simulink model "H175_Anode_Integration"  (R2023a)
settings: Solver=VariableStepAuto  StartTime=0.0  StopTime=80  RelTol=1e-3
values from neighbouring files (symbols this model uses):
  anode_tube_D = 0.01    [All_Properties.mat]    (also in anode_subsystem_parameters.m; environment_parameters.m)
  D = 0.01    [All_Properties.mat]    (also in anode_subsystem_parameters.m)
  densityHydrogen = 0.0899    [All_Properties.mat]    (also in Valve_Init.m; anode_subsystem_parameters.m)
  Kv_VL6112 = 0.8    [All_Properties.mat]    (also in anode_subsystem_parameters.m)
  N2_T = [-56.55 -50 -40 -30 -20 -10 -5 -4 -3 -2 -1 0 ... (52 elements, 1x52)]    [All_Properties.mat]    (also in anode_subsystem_parameters.m = [-56.55 -50 -40 -30 -20 -10 -5 -4 -3 -2 -1 0 1 2 3 4 5 10 20; environment_parameters.m = [-56.55, -50:10:-10, -5:1:5, 10:10:350]; stack_model_harness_parameters.m = [-56.55, -50:10:-10, -5:1:5, 10:10:350])
  p_range = 0.005    [All_Properties.mat]    (also in anode_subsystem_parameters.m)
  r_max = 0.2    [All_Properties.mat]    (also in anode_subsystem_parameters.m)
  r_min = 0.0001    [All_Properties.mat]    (also in anode_subsystem_parameters.m)
  responseTimeValve = 0.013    [All_Properties.mat]    (also in anode_subsystem_parameters.m)
libraries: fl_lib x75, nesl_utility x39, SimscapeFluids_lib x1
(part 2 of 2)

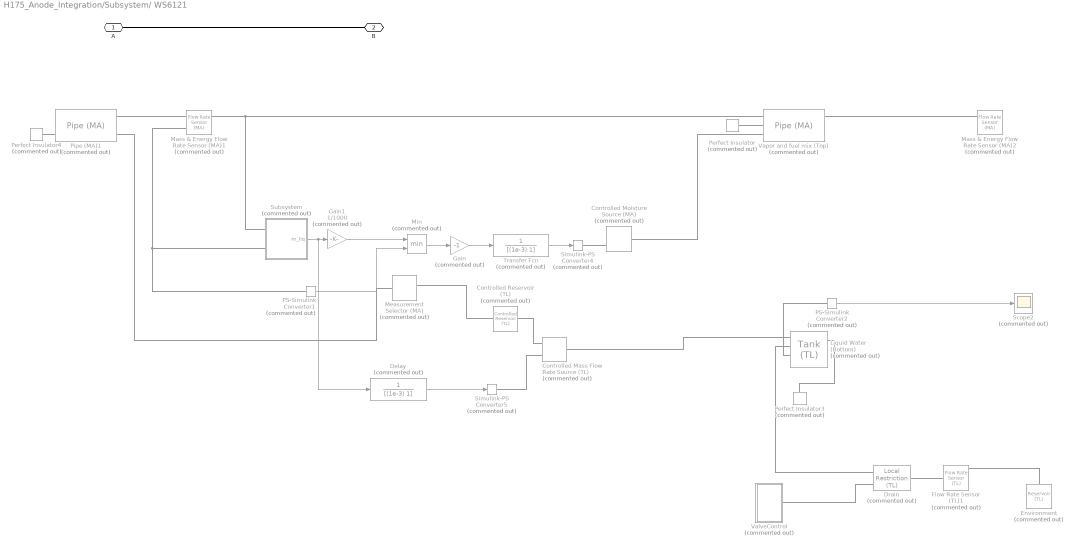
== system H175_Anode_Integration/Subsystem/ WS6121 ==
  Controlled Mass Flow Rate Source (TL) : fl_lib/Thermal Liquid/Sources/Controlled Mass Flow Rate Source (TL)  Commented=on  power_spec=foundation.enum.power_spec.isentropic  area=0.01 m^2
      settings: InternalSimscapePortConfiguration="{\"Bottom\":[],\"Left\":[{\"id\":\"A\",\"label\":\"A\",\"type\":\"foundation.thermal_liquid.thermal_liquid\"},{\"id\":\"M\",\"label\":\"M\",\"type\":\"input\"}],\"Right\":[{\"id\":\"B\",\"label\":\"B\",\"type\":\"foundation.thermal_liquid.thermal_liquid\"}],\"Top\":[]}"
  Controlled Moisture Source (MA) : fl_lib/Moist Air/Sources/Moisture & Trace Gas Sources/Controlled Moisture Source (MA)  Commented=on  moisture_source_spec=foundation.enum.moisture_source_spec.liquid  Phi_S_specify=off  Phi_S_priority=None  Phi_S=0 kW  Phi_S_nominal_specify=off  Phi_S_nominal_unit=kW  Phi_S_nominal_value=1  mdot_w_S_specify=off  mdot_w_S_priority=None  mdot_w_S=0 kg/s  mdot_w_S_nominal_specify=off  mdot_w_S_nominal_unit=kg/s  mdot_w_S_nominal_value=1
      settings: InternalSimscapePortConfiguration="{\"Bottom\":[],\"Left\":[{\"id\":\"S\",\"label\":\"S\",\"type\":\"foundation.moist_air.moist_air_source\"}],\"Right\":[{\"id\":\"M\",\"label\":\"M\",\"type\":\"input\"},{\"id\":\"T\",\"label\":\"T\",\"type\":\"input\"}],\"Top\":[]}"
  Controlled Reservoir (TL) : fl_lib/Thermal Liquid/Elements/Controlled Reservoir (TL)  Commented=on  pressure_spec=foundation.enum.pressure_spec.atmospheric  reservoir_pressure=0.101325 MPa  area=0.01 m^2
      settings: InternalSimscapePortConfiguration="{\"Bottom\":[],\"Left\":[{\"id\":\"A\",\"label\":\"A\",\"type\":\"foundation.thermal_liquid.thermal_liquid\"}],\"Right\":[{\"id\":\"T_in\",\"label\":\"T\",\"type\":\"input\"}],\"Top\":[]}"
  Delay : TransferFcn  Commented=on  Denominator=[(1e-3) 1]
  Drain : fl_lib/Thermal Liquid/Elements/Local Restriction (TL)  Commented=on  restriction_type=foundation.enum.restriction_type.variable  restriction_area=0.001 m^2  min_area=0.00001e-6 m^2  max_area=4.75e-6 m^2  area=0.00358 m^2  Cd=0.32  Re_c=150  pressure_recovery=simscape.enum.onoff.off
      settings: InternalSimscapePortConfiguration="{\"Bottom\":[],\"Left\":[{\"id\":\"A\",\"label\":\"A\",\"type\":\"foundation.thermal_liquid.thermal_liquid\"},{\"id\":\"area_in\",\"label\":\"AR\",\"type\":\"input\"}],\"Right\":[{\"id\":\"B\",\"label\":\"B\",\"type\":\"foundation.thermal_liquid.thermal_liquid\"}],\"Top\":[]}"
  Environment : fl_lib/Thermal Liquid/Elements/Reservoir (TL)  Commented=on  pressure_spec=foundation.enum.pressure_spec.atmospheric  reservoir_pressure=0.101325 MPa  reservoir_temperature=293.15 K  area=0.01 m^2
  Flow Rate Sensor (TL)1 : fl_lib/Thermal Liquid/Sensors/Flow Rate Sensor (TL)  Commented=on  mass_flow_measure=true  volumetric_flow_measure=false  energy_flow_measure=true
      settings: InternalSimscapePortConfiguration="{\"Bottom\":[{\"id\":\"PHI\",\"label\":\"φ\",\"type\":\"output\"}],\"Left\":[{\"id\":\"A\",\"label\":\"A\",\"type\":\"foundation.thermal_liquid.thermal_liquid\"}],\"Right\":[{\"id\":\"B\",\"label\":\"B\",\"type\":\"foundation.thermal_liquid.thermal_liquid\"},{\"id\":\"M\",\"label\":\"M\",\"type\":\"output\"}],\"Top\":[]}"
  Gain : Gain  Commented=on  Gain=-1
  Gain1 : Gain  Commented=on  Gain=1/1000
  "Liquid Water (Bottom) " : SimscapeFluids_lib/Thermal Liquid/Tanks & Accumulators/Tank (TL)  Commented=on  num_inlet=fluids.thermal_liquid.tanks_accumulators.enum.NumInlet.Two  pressure_spec=foundation.enum.pressure_spec.atmospheric  tank_pressure=0.101325 MPa  volume_spec=fluids.thermal_liquid.tanks_accumulators.enum.TankVolumeSpec.Constant  tank_area=0.0003 m^2  level_TLU=[0, 3, 5] m  volume_TLU=[0, 4, 6] m^3  inlet_height_A=0.00002 m  inlet_area_A=0.00002 m^2  inlet_heights_AB=[.1, .1] m  inlet_areas_AB=[.01, .01] m^2  inlet_heights_ABC=[.1, .1, .1] m  inlet_areas_ABC=[.01, .01, .01] m^2  inlet_heights_ABCD=0.1 * ones(1, 4) m  inlet_areas_ABCD=0.01 * ones(1, 4) m^2  inlet_heights_ABCDE=0.1 * ones(1, 5) m  inlet_areas_ABCDE=0.01 * ones(1, 5) m^2  inlet_heights_ABCDEF=0.1 * ones(1, 6) m  inlet_areas_ABCDEF=0.01 * ones(1, 6) m^2  level_check=simscape.enum.assert.action.error  capacity_check=simscape.enum.assert.action.warn  max_capacity=0.0003 m^3  g=9.81 m/s^2  level_specify=off  level_priority=High  level=5 m  level_nominal_specify=off  level_nominal_unit=m  level_nominal_value=1  volume_specify=off  volume_priority=None  volume=5 m^3  volume_nominal_specify=off  volume_nominal_unit=m^3  volume_nominal_value=1  mass_specify=off  mass_priority=None  mass=5000 kg  mass_nominal_specify=off  mass_nominal_unit=kg  mass_nominal_value=1  T_I_specify=off  T_I_priority=High  T_I=293.15 K  T_I_nominal_specify=off  T_I_nominal_unit=K  T_I_nominal_value=1
      settings: InternalSimscapePortConfiguration="{\"Bottom\":[{\"id\":\"H\",\"label\":\"H\",\"type\":\"foundation.thermal.thermal\"},{\"id\":\"T_out\",\"label\":\"T\",\"type\":\"output\"}],\"Left\":[{\"id\":\"A\",\"label\":\"A\",\"type\":\"foundation.thermal_liquid.thermal_liquid\"},{\"id\":\"B\",\"label\":\"B\",\"type\":\"foundation.thermal_liquid.thermal_liquid\"}],\"Right\":[],\"Top\":[{\"id\":\"V_out\",\"label\":\"V\",\"type\":\"output\"},{\"id\":\"L_out\",\"label\":\"L\",\"type\":\"output\"}]}"
  Mass & Energy Flow Rate Sensor (MA)1 : fl_lib/Moist Air/Sensors/Flow Rate Sensor (MA)  Commented=on  mass_flow_measure=true  volumetric_flow_measure=false  volumetric_flow_conditions=foundation.enum.volumetric_flow_conditions.actual  p_std=0.101325 MPa  T_std=20 degC  RH_std=0.65  energy_flow_measure=false  vapor_flow_measure=true  gas_flow_measure=false
      settings: InternalSimscapePortConfiguration="{\"Bottom\":[],\"Left\":[{\"id\":\"A\",\"label\":\"A\",\"type\":\"foundation.moist_air.moist_air\"},{\"id\":\"Mw\",\"label\":\"Mw\",\"type\":\"output\"}],\"Right\":[{\"id\":\"B\",\"label\":\"B\",\"type\":\"foundation.moist_air.moist_air\"},{\"id\":\"M\",\"label\":\"M\",\"type\":\"output\"}],\"Top\":[]}"
  Mass & Energy Flow Rate Sensor (MA)2 : fl_lib/Moist Air/Sensors/Flow Rate Sensor (MA)  Commented=on  mass_flow_measure=true  volumetric_flow_measure=false  volumetric_flow_conditions=foundation.enum.volumetric_flow_conditions.actual  p_std=0.101325 MPa  T_std=20 degC  RH_std=0.65  energy_flow_measure=false  vapor_flow_measure=true  gas_flow_measure=false
      settings: InternalSimscapePortConfiguration="{\"Bottom\":[],\"Left\":[{\"id\":\"A\",\"label\":\"A\",\"type\":\"foundation.moist_air.moist_air\"},{\"id\":\"Mw\",\"label\":\"Mw\",\"type\":\"output\"}],\"Right\":[{\"id\":\"B\",\"label\":\"B\",\"type\":\"foundation.moist_air.moist_air\"},{\"id\":\"M\",\"label\":\"M\",\"type\":\"output\"}],\"Top\":[]}"
  Measurement Selector (MA) : fl_lib/Moist Air/Sensors/Measurement Selector (MA)  Commented=on  moisture_spec=foundation.enum.moisture_spec.relative_humidity  trace_gas_spec=foundation.enum.trace_gas_spec.mass_fraction
  Min : MinMax  Commented=on  Inputs=2
  PS-Simulink Converter1 : nesl_utility/PS-Simulink Converter  Commented=on  PhysicalDomain=network_engine_domain  SubClassName=ps_output  LeftPortType=input  RightPortType=output  PseudoPeriodic=off  Frequencies=[]  VectorFormat=inherit  Unit=inherit  AffineConversion=off
  PS-Simulink Converter2 : nesl_utility/PS-Simulink Converter  Commented=on  PhysicalDomain=network_engine_domain  SubClassName=ps_output  LeftPortType=input  RightPortType=output  PseudoPeriodic=off  Frequencies=[]  VectorFormat=inherit  Unit=inherit  AffineConversion=off
  Perfect Insulator : fl_lib/Thermal/Thermal Elements/Perfect Insulator  Commented=on  T_specify=off  T_priority=None  T=0 K  T_nominal_specify=off  T_nominal_unit=K  T_nominal_value=1
  Perfect Insulator3 : fl_lib/Thermal/Thermal Elements/Perfect Insulator  Commented=on  T_specify=off  T_priority=None  T=293.15 K  T_nominal_specify=off  T_nominal_unit=K  T_nominal_value=1
  Perfect Insulator4 : fl_lib/Thermal/Thermal Elements/Perfect Insulator  Commented=on  T_specify=off  T_priority=None  T=0 K  T_nominal_specify=off  T_nominal_unit=K  T_nominal_value=1
  Pipe (MA)1 : fl_lib/Moist Air/Elements/Pipe (MA)  Commented=on  length=0.25 m  area=pi*0.05^2/4 m^2  Dh=0.05 m  length_add=0.1 m  roughness=15e-6 m  Re_lam=2000  Re_tur=4000  shape_factor=64  Nu_lam=3.66  wall_condensation=simscape.enum.onoff.off  RH_ws=1  time_constant=1e-3 s  moisture_trace_gas_source=foundation.enum.moisture_trace_gas_source.none  moisture_source_spec=foundation.enum.moisture_source_spec.vapor  moisture_mass_flow=0 kg/s  moisture_temperature_spec=foundation.enum.temperature_spec.atmospheric  moisture_temperature=293.15 K  trace_gas_mass_flow=0 kg/s  trace_gas_temperature_spec=foundation.enum.temperature_spec.atmospheric  trace_gas_temperature=293.15 K  p_I_specify=on  p_I_priority=High  p_I=env_p MPa  p_I_nominal_specify=off  p_I_nominal_unit=MPa  p_I_nominal_value=1  T_I_specify=on  T_I_priority=High  T_I=env_T degC  T_I_nominal_specify=off  T_I_nominal_unit=K  T_I_nominal_value=1  RH_I_specify=off  RH_I_priority=High  RH_I=0  RH_I_nominal_specify=off  RH_I_nominal_unit=1  RH_I_nominal_value=1  x_w_I_specify=off  x_w_I_priority=None  x_w_I=0  x_w_I_nominal_specify=off  x_w_I_nominal_unit=1  x_w_I_nominal_value=1  y_w_I_specify=off  y_w_I_priority=None  y_w_I=0  y_w_I_nominal_specify=off  y_w_I_nominal_unit=1  y_w_I_nominal_value=1  HR_I_specify=off  HR_I_priority=None  HR_I=0  HR_I_nominal_specify=off  HR_I_nominal_unit=1  HR_I_nominal_value=1  x_g_I_specify=on  x_g_I_priority=None  x_g_I=0  x_g_I_nominal_specify=off  x_g_I_nominal_unit=1  x_g_I_nominal_value=1  y_g_I_specify=on  y_g_I_priority=High  y_g_I=tank_yH2  y_g_I_nominal_specify=off  y_g_I_nominal_unit=1  y_g_I_nominal_value=1
  Scope2 : Scope  Commented=on
  Simulink-PS Converter4 : nesl_utility/Simulink-PS Converter  Commented=on  PhysicalDomain=network_engine_domain  SubClassName=ps_input  LeftPortType=input  RightPortType=output  PseudoPeriodic=off  Frequencies=[]  NoiseDistribution=none  NoiseParameters=[]  Unit=1  AffineConversion=off  FilteringAndDerivatives=provide  SimscapeFilterOrder=1  InputFilterTimeConstant=0.001  UdotUserProvided=0
  Simulink-PS Converter5 : nesl_utility/Simulink-PS Converter  Commented=on  PhysicalDomain=network_engine_domain  SubClassName=ps_input  LeftPortType=input  RightPortType=output  PseudoPeriodic=off  Frequencies=[]  NoiseDistribution=none  NoiseParameters=[]  Unit=1  AffineConversion=off  FilteringAndDerivatives=provide  SimscapeFilterOrder=1  InputFilterTimeConstant=0.001  UdotUserProvided=0
  Subsystem : Subsystem  Commented=on
  Transfer Fcn : TransferFcn  Commented=on  Denominator=[(1e-3) 1]
  ValveControl : Subsystem  Commented=on
  Vapor and fuel mix (Top) : fl_lib/Moist Air/Elements/Pipe (MA)  Commented=on  length=0.25 m  area=pi*0.05^2/4 m^2  Dh=0.05 m  length_add=0.1 m  roughness=15e-6 m  Re_lam=2000  Re_tur=4000  shape_factor=64  Nu_lam=3.66  wall_condensation=simscape.enum.onoff.off  RH_ws=1  time_constant=1e-3 s  moisture_trace_gas_source=foundation.enum.moisture_trace_gas_source.controlled  moisture_source_spec=foundation.enum.moisture_source_spec.vapor  moisture_mass_flow=0 kg/s  moisture_temperature_spec=foundation.enum.temperature_spec.atmospheric  moisture_temperature=293.15 K  trace_gas_mass_flow=0 kg/s  trace_gas_temperature_spec=foundation.enum.temperature_spec.atmospheric  trace_gas_temperature=293.15 K  p_I_specify=on  p_I_priority=High  p_I=env_p MPa  p_I_nominal_specify=off  p_I_nominal_unit=MPa  p_I_nominal_value=1  T_I_specify=on  T_I_priority=High  T_I=env_T degC  T_I_nominal_specify=off  T_I_nominal_unit=K  T_I_nominal_value=1  RH_I_specify=off  RH_I_priority=High  RH_I=0  RH_I_nominal_specify=off  RH_I_nominal_unit=1  RH_I_nominal_value=1  x_w_I_specify=off  x_w_I_priority=None  x_w_I=0  x_w_I_nominal_specify=off  x_w_I_nominal_unit=1  x_w_I_nominal_value=1  y_w_I_specify=off  y_w_I_priority=None  y_w_I=0  y_w_I_nominal_specify=off  y_w_I_nominal_unit=1  y_w_I_nominal_value=1  HR_I_specify=off  HR_I_priority=None  HR_I=0  HR_I_nominal_specify=off  HR_I_nominal_unit=1  HR_I_nominal_value=1  x_g_I_specify=on  x_g_I_priority=None  x_g_I=0  x_g_I_nominal_specify=off  x_g_I_nominal_unit=1  x_g_I_nominal_value=1  y_g_I_specify=on  y_g_I_priority=High  y_g_I=tank_yH2  y_g_I_nominal_specify=off  y_g_I_nominal_unit=1  y_g_I_nominal_value=1
      settings: InternalSimscapePortConfiguration="{\"Bottom\":[],\"Left\":[{\"id\":\"A\",\"label\":\"A\",\"type\":\"foundation.moist_air.moist_air\"},{\"id\":\"H\",\"label\":\"H\",\"type\":\"foundation.thermal.thermal\"},{\"id\":\"S\",\"label\":\"S\",\"type\":\"foundation.moist_air.moist_air_source\"}],\"Right\":[{\"id\":\"B\",\"label\":\"B\",\"type\":\"foundation.moist_air.moist_air\"},{\"id\":\"W\",\"label\":\"W\",\"type\":\"output\"},{\"id\":\"F\",\"label\":\"F\",\"type\":\"output\"}],\"Top\":[]}"
  A : PMIOPort  Side=Left
  B : PMIOPort  Port=2  Side=Right
  wires:
  Delay/1 -> Simulink-PS Converter5/1
  PS-Simulink Converter1/1 -> Min/2
  Gain1/1 -> Min/1
  Min/1 -> Gain/1
  Transfer Fcn/1 -> Simulink-PS Converter4/1
  Gain/1 -> Transfer Fcn/1
  Subsystem/1(m_liq) -> Delay/1, Gain1/1
  PS-Simulink Converter2/1 -> Scope2/1
  connections:
  Perfect Insulator/LConn1 -- Vapor and fuel mix (Top)/LConn2
  Controlled Reservoir (TL)/RConn1 -- Measurement Selector (MA)/RConn2
  Controlled Mass Flow Rate Source (TL)/LConn1 -- Controlled Reservoir (TL)/LConn1
  Simulink-PS Converter5/RConn1 -- Controlled Mass Flow Rate Source (TL)/LConn2
  Simulink-PS Converter4/RConn1 -- Controlled Moisture Source (MA)/RConn1
  "Liquid Water (Bottom) "/LConn1 -- Controlled Mass Flow Rate Source (TL)/RConn1
  Perfect Insulator3/LConn1 -- "Liquid Water (Bottom) "/RConn1
  PS-Simulink Converter2/LConn1 -- "Liquid Water (Bottom) "/LConn3
  Mass & Energy Flow Rate Sensor (MA)2/LConn1 -- Vapor and fuel mix (Top)/RConn1
  Mass & Energy Flow Rate Sensor (MA)1/RConn1 -- Subsystem/LConn1 -- Vapor and fuel mix (Top)/LConn1
  Subsystem/LConn2 -- PS-Simulink Converter1/LConn1 -- Mass & Energy Flow Rate Sensor (MA)1/LConn2
  Controlled Moisture Source (MA)/LConn1 -- Vapor and fuel mix (Top)/LConn3
  Perfect Insulator4/LConn1 -- Pipe (MA)1/LConn2
  Pipe (MA)1/RConn1 -- Mass & Energy Flow Rate Sensor (MA)1/LConn1
  Pipe (MA)1/RConn3 -- Measurement Selector (MA)/LConn1
  Drain/LConn1 -- "Liquid Water (Bottom) "/LConn2
  Drain/RConn1 -- Flow Rate Sensor (TL)1/LConn1
  Flow Rate Sensor (TL)1/RConn1 -- Environment/LConn1
  ValveControl/RConn1 -- Drain/LConn2
  A/RConn1 -- B/RConn1

== system H175_Anode_Integration/Subsystem/S1a ==
  Flow Rate Sensor (MA) : fl_lib/Moist Air/Sensors/Flow Rate Sensor (MA)  mass_flow_measure=true  volumetric_flow_measure=false  volumetric_flow_conditions=foundation.enum.volumetric_flow_conditions.actual  p_std=0.101325 MPa  T_std=20 degC  RH_std=0.65  energy_flow_measure=true  vapor_flow_measure=false  gas_flow_measure=false
      settings: InternalSimscapePortConfiguration="{\"Bottom\":[{\"id\":\"PHI\",\"label\":\"φ\",\"type\":\"output\"}],\"Left\":[{\"id\":\"A\",\"label\":\"A\",\"type\":\"foundation.moist_air.moist_air\"}],\"Right\":[{\"id\":\"B\",\"label\":\"B\",\"type\":\"foundation.moist_air.moist_air\"},{\"id\":\"M\",\"label\":\"M\",\"type\":\"output\"}],\"Top\":[]}"
  Gain1 : Gain  Gain=1000
  PS-Simulink Converter2 : nesl_utility/PS-Simulink Converter  PhysicalDomain=network_engine_domain  SubClassName=ps_output  LeftPortType=input  RightPortType=output  PseudoPeriodic=off  Frequencies=[]  VectorFormat=inherit  Unit=inherit  AffineConversion=off
  PS-Simulink Converter3 : nesl_utility/PS-Simulink Converter  PhysicalDomain=network_engine_domain  SubClassName=ps_output  LeftPortType=input  RightPortType=output  PseudoPeriodic=off  Frequencies=[]  VectorFormat=inherit  Unit=inherit  AffineConversion=off
  Pressure & Temperature Sensor (MA) : fl_lib/Moist Air/Sensors/Pressure & Temperature Sensor (MA)  reference=foundation.enum.MeasurementReference.absolute  pressure=true  pressure_spec=foundation.enum.PressureMeasementSpec.Absolute  temperature=false
      settings: InternalSimscapePortConfiguration="{\"Bottom\":[],\"Left\":[{\"id\":\"A\",\"label\":\"A\",\"type\":\"foundation.moist_air.moist_air\"}],\"Right\":[{\"id\":\"Pa\",\"label\":\"Pa\",\"type\":\"output\"}],\"Top\":[]}"
  To Workspace : ToWorkspace  VariableName=mdot_H2  SaveFormat=Structure With Time  SampleTime=-1
  To Workspace1 : ToWorkspace  VariableName=Pressure_Tank  SaveFormat=Structure With Time  SampleTime=-1
  A : PMIOPort  Side=Left
  B : PMIOPort  Port=2  Side=Right
  wires:
  Gain1/1 -> To Workspace/1
  PS-Simulink Converter3/1 -> Gain1/1
  PS-Simulink Converter2/1 -> To Workspace1/1
  connections:
  PS-Simulink Converter2/LConn1 -- Pressure & Temperature Sensor (MA)/RConn1
  Pressure & Temperature Sensor (MA)/LConn1 -- A/RConn1 -- Flow Rate Sensor (MA)/LConn1
  Flow Rate Sensor (MA)/RConn2 -- PS-Simulink Converter3/LConn1
  Flow Rate Sensor (MA)/RConn1 -- B/RConn1

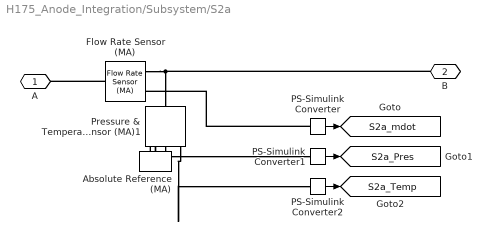
== system H175_Anode_Integration/Subsystem/S2a ==
  Absolute Reference (MA) : fl_lib/Moist Air/Elements/Absolute Reference (MA)
  Flow Rate Sensor (MA) : fl_lib/Moist Air/Sensors/Flow Rate Sensor (MA)  mass_flow_measure=true  volumetric_flow_measure=false  volumetric_flow_conditions=foundation.enum.volumetric_flow_conditions.actual  p_std=0.101325 MPa  T_std=20 degC  RH_std=0.65  energy_flow_measure=false  vapor_flow_measure=false  gas_flow_measure=false
      settings: LogSimulationData=on  InternalSimscapePortConfiguration="{\"Bottom\":[],\"Left\":[{\"id\":\"A\",\"label\":\"A\",\"type\":\"foundation.moist_air.moist_air\"}],\"Right\":[{\"id\":\"B\",\"label\":\"B\",\"type\":\"foundation.moist_air.moist_air\"},{\"id\":\"M\",\"label\":\"M\",\"type\":\"output\"}],\"Top\":[]}"
  PS-Simulink Converter : nesl_utility/PS-Simulink Converter  PhysicalDomain=network_engine_domain  SubClassName=ps_output  LeftPortType=input  RightPortType=output  PseudoPeriodic=off  Frequencies=[]  VectorFormat=inherit  Unit=inherit  AffineConversion=off
  PS-Simulink Converter1 : nesl_utility/PS-Simulink Converter  PhysicalDomain=network_engine_domain  SubClassName=ps_output  LeftPortType=input  RightPortType=output  PseudoPeriodic=off  Frequencies=[]  VectorFormat=inherit  Unit=inherit  AffineConversion=off
  PS-Simulink Converter2 : nesl_utility/PS-Simulink Converter  PhysicalDomain=network_engine_domain  SubClassName=ps_output  LeftPortType=input  RightPortType=output  PseudoPeriodic=off  Frequencies=[]  VectorFormat=inherit  Unit=inherit  AffineConversion=off
  Pressure & Temperature Sensor (MA)1 : fl_lib/Moist Air/Sensors/Pressure & Temperature Sensor (MA)  reference=foundation.enum.MeasurementReference.difference  pressure=true  pressure_spec=foundation.enum.PressureMeasementSpec.Absolute  temperature=true
      settings: InternalSimscapePortConfiguration="{\"Bottom\":[{\"id\":\"T\",\"label\":\"T\",\"type\":\"output\"}],\"Left\":[{\"id\":\"A\",\"label\":\"A\",\"type\":\"foundation.moist_air.moist_air\"}],\"Right\":[{\"id\":\"B\",\"label\":\"B\",\"type\":\"foundation.moist_air.moist_air\"},{\"id\":\"P\",\"label\":\"P\",\"type\":\"output\"}],\"Top\":[]}"
  A : PMIOPort  Side=Left
  B : PMIOPort  Port=2  Side=Right
  tag scope: S2a_Pres=global, S2a_Temp=global, S2a_mdot=global
  wires:
  PS-Simulink Converter/1 -> [S2a_mdot]
  PS-Simulink Converter1/1 -> [S2a_Pres]
  PS-Simulink Converter2/1 -> [S2a_Temp]
  connections:
  Flow Rate Sensor (MA)/RConn1 -- B/RConn1 -- Pressure & Temperature Sensor (MA)1/LConn1
  Pressure & Temperature Sensor (MA)1/RConn2 -- PS-Simulink Converter1/LConn1
  Pressure & Temperature Sensor (MA)1/RConn3 -- PS-Simulink Converter2/LConn1
  Flow Rate Sensor (MA)/LConn1 -- A/RConn1
  Absolute Reference (MA)/LConn1 -- Pressure & Temperature Sensor (MA)1/RConn1
  PS-Simulink Converter/LConn1 -- Flow Rate Sensor (MA)/RConn2

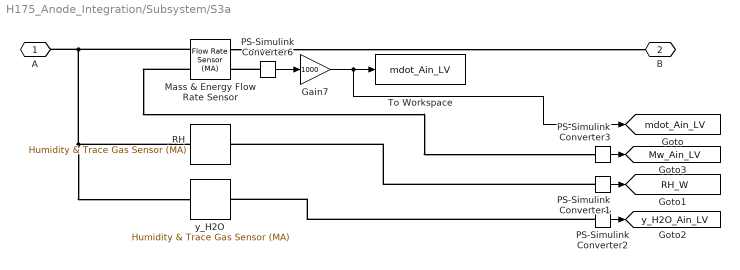
== system H175_Anode_Integration/Subsystem/S3a ==
  Gain7 : Gain  Gain=1000
  "Mass & Energy Flow Rate Sensor " : fl_lib/Moist Air/Sensors/Flow Rate Sensor (MA)  mass_flow_measure=true  volumetric_flow_measure=false  volumetric_flow_conditions=foundation.enum.volumetric_flow_conditions.actual  p_std=0.101325 MPa  T_std=20 degC  RH_std=0.65  energy_flow_measure=false  vapor_flow_measure=true  gas_flow_measure=false
      settings: InternalSimscapePortConfiguration="{\"Bottom\":[],\"Left\":[{\"id\":\"A\",\"label\":\"A\",\"type\":\"foundation.moist_air.moist_air\"},{\"id\":\"Mw\",\"label\":\"Mw\",\"type\":\"output\"}],\"Right\":[{\"id\":\"B\",\"label\":\"B\",\"type\":\"foundation.moist_air.moist_air\"},{\"id\":\"M\",\"label\":\"M\",\"type\":\"output\"}],\"Top\":[]}"
  PS-Simulink Converter{1..3,6} (4 alike) : nesl_utility/PS-Simulink Converter  PhysicalDomain=network_engine_domain  SubClassName=ps_output  LeftPortType=input  RightPortType=output  PseudoPeriodic=off  Frequencies=[]  VectorFormat=inherit  Unit=inherit  AffineConversion=off
  RH : fl_lib/Moist Air/Sensors/Humidity & Trace Gas Sensor (MA)  moisture_on=true  moisture_spec=foundation.enum.moistureSpec.RelativeHumidity  trace_gas_on=false  trace_gas_spec=foundation.enum.trace_gas_spec.mole_fraction
      settings: InternalSimscapePortConfiguration="{\"Bottom\":[],\"Left\":[{\"id\":\"A\",\"label\":\"A\",\"type\":\"foundation.moist_air.moist_air\"}],\"Right\":[{\"id\":\"W\",\"label\":\"W\",\"type\":\"output\"}],\"Top\":[]}"
  To Workspace : ToWorkspace  VariableName=mdot_Ain_LV  SaveFormat=Structure With Time  SampleTime=-1
  y_H2O : fl_lib/Moist Air/Sensors/Humidity & Trace Gas Sensor (MA)  moisture_on=true  moisture_spec=foundation.enum.moistureSpec.MoleFraction  trace_gas_on=false  trace_gas_spec=foundation.enum.trace_gas_spec.mole_fraction
      settings: InternalSimscapePortConfiguration="{\"Bottom\":[],\"Left\":[{\"id\":\"A\",\"label\":\"A\",\"type\":\"foundation.moist_air.moist_air\"}],\"Right\":[{\"id\":\"W\",\"label\":\"W\",\"type\":\"output\"}],\"Top\":[]}"
  A : PMIOPort  Side=Left
  B : PMIOPort  Port=2  Side=Right
  tag scope: Mw_Ain_LV=global, RH_W=global, mdot_Ain_LV=global, y_H2O_Ain_LV=global
  wires:
  PS-Simulink Converter6/1 -> Gain7/1
  Gain7/1 -> [mdot_Ain_LV], To Workspace/1
  PS-Simulink Converter1/1 -> [RH_W]
  PS-Simulink Converter2/1 -> [y_H2O_Ain_LV]
  PS-Simulink Converter3/1 -> [Mw_Ain_LV]
  connections:
  RH/LConn1 -- y_H2O/LConn1 -- A/RConn1 -- "Mass & Energy Flow Rate Sensor "/LConn1
  PS-Simulink Converter6/LConn1 -- "Mass & Energy Flow Rate Sensor "/RConn2
  "Mass & Energy Flow Rate Sensor "/RConn1 -- B/RConn1
  PS-Simulink Converter2/LConn1 -- y_H2O/RConn1
  "Mass & Energy Flow Rate Sensor "/LConn2 -- PS-Simulink Converter3/LConn1
  PS-Simulink Converter1/LConn1 -- RH/RConn1

== system H175_Anode_Integration/Subsystem/S4a ==
  Anodein_mdot : fl_lib/Moist Air/Sensors/Flow Rate Sensor (MA)  mass_flow_measure=true  volumetric_flow_measure=false  volumetric_flow_conditions=foundation.enum.volumetric_flow_conditions.actual  p_std=0.101325 MPa  T_std=20 degC  RH_std=0.65  energy_flow_measure=false  vapor_flow_measure=true  gas_flow_measure=false
      settings: InternalSimscapePortConfiguration="{\"Bottom\":[],\"Left\":[{\"id\":\"A\",\"label\":\"A\",\"type\":\"foundation.moist_air.moist_air\"},{\"id\":\"Mw\",\"label\":\"Mw\",\"type\":\"output\"}],\"Right\":[{\"id\":\"B\",\"label\":\"B\",\"type\":\"foundation.moist_air.moist_air\"},{\"id\":\"M\",\"label\":\"M\",\"type\":\"output\"}],\"Top\":[]}"
  Gain8 : Gain  Gain=1000
  PS-Simulink Converter7 : nesl_utility/PS-Simulink Converter  PhysicalDomain=network_engine_domain  SubClassName=ps_output  LeftPortType=input  RightPortType=output  PseudoPeriodic=off  Frequencies=[]  VectorFormat=inherit  Unit=inherit  AffineConversion=off
  To Workspace2 : ToWorkspace  VariableName=mdot_Ain_V  SaveFormat=Structure With Time  SampleTime=-1
  B : PMIOPort  Side=Right
  A : PMIOPort  Port=2  Side=Left
  wires:
  PS-Simulink Converter7/1 -> Gain8/1
  Gain8/1 -> To Workspace2/1
  connections:
  Anodein_mdot/LConn1 -- A/RConn1
  PS-Simulink Converter7/LConn1 -- Anodein_mdot/RConn2
  Anodein_mdot/RConn1 -- B/RConn1

== system H175_Anode_Integration/Subsystem/S5a ==
  Constant : Constant  Value=343
  Controlled Reservoir (MA) : fl_lib/Moist Air/Elements/Controlled Reservoir (MA)  moisture_spec=foundation.enum.moistureSpec.RelativeHumidity  trace_gas_spec=foundation.enum.trace_gas_spec.mass_fraction  RH_ws=1  area_A=0.01 m^2  input_error_spec=foundation.enum.input_range_error.warn
      settings: InternalSimscapePortConfiguration="{\"Bottom\":[],\"Left\":[{\"id\":\"A\",\"label\":\"A\",\"type\":\"foundation.moist_air.moist_air\"}],\"Right\":[{\"id\":\"T\",\"label\":\"T\",\"type\":\"input\"},{\"id\":\"P\",\"label\":\"P\",\"type\":\"input\"},{\"id\":\"W\",\"label\":\"W\",\"type\":\"input\"},{\"id\":\"G\",\"label\":\"G\",\"type\":\"input\"}],\"Top\":[]}"
  Flow Rate Sensor (MA) : fl_lib/Moist Air/Sensors/Flow Rate Sensor (MA)  mass_flow_measure=true  volumetric_flow_measure=false  volumetric_flow_conditions=foundation.enum.volumetric_flow_conditions.actual  p_std=0.101325 MPa  T_std=20 degC  RH_std=0.65  energy_flow_measure=false  vapor_flow_measure=false  gas_flow_measure=false
      settings: InternalSimscapePortConfiguration="{\"Bottom\":[],\"Left\":[{\"id\":\"A\",\"label\":\"A\",\"type\":\"foundation.moist_air.moist_air\"}],\"Right\":[{\"id\":\"B\",\"label\":\"B\",\"type\":\"foundation.moist_air.moist_air\"},{\"id\":\"M\",\"label\":\"M\",\"type\":\"output\"}],\"Top\":[]}"
  Flow Rate Sensor (MA)1 : fl_lib/Moist Air/Sensors/Flow Rate Sensor (MA)  mass_flow_measure=true  volumetric_flow_measure=false  volumetric_flow_conditions=foundation.enum.volumetric_flow_conditions.actual  p_std=0.101325 MPa  T_std=20 degC  RH_std=0.65  energy_flow_measure=false  vapor_flow_measure=false  gas_flow_measure=false
      settings: InternalSimscapePortConfiguration="{\"Bottom\":[],\"Left\":[{\"id\":\"A\",\"label\":\"A\",\"type\":\"foundation.moist_air.moist_air\"}],\"Right\":[{\"id\":\"B\",\"label\":\"B\",\"type\":\"foundation.moist_air.moist_air\"},{\"id\":\"M\",\"label\":\"M\",\"type\":\"output\"}],\"Top\":[]}"
  Simulink-PS Converter : nesl_utility/Simulink-PS Converter  PhysicalDomain=network_engine_domain  SubClassName=ps_input  LeftPortType=input  RightPortType=output  PseudoPeriodic=off  Frequencies=[]  NoiseDistribution=none  NoiseParameters=[]  Unit=bar  AffineConversion=off  FilteringAndDerivatives=provide  SimscapeFilterOrder=1  InputFilterTimeConstant=0.001  UdotUserProvided=0
  Simulink-PS Converter1 : nesl_utility/Simulink-PS Converter  PhysicalDomain=network_engine_domain  SubClassName=ps_input  LeftPortType=input  RightPortType=output  PseudoPeriodic=off  Frequencies=[]  NoiseDistribution=none  NoiseParameters=[]  Unit=K  AffineConversion=off  FilteringAndDerivatives=provide  SimscapeFilterOrder=1  InputFilterTimeConstant=0.001  UdotUserProvided=0
  B : PMIOPort  Side=Left
  A : PMIOPort  Port=2  Side=Right
  wires:
  [p_Desired] -> Simulink-PS Converter/1
  Constant/1 -> Simulink-PS Converter1/1
  connections:
  A/RConn1 -- Flow Rate Sensor (MA)/LConn1
  Controlled Reservoir (MA)/LConn1 -- Flow Rate Sensor (MA)1/LConn1 -- Flow Rate Sensor (MA)/RConn1
  Simulink-PS Converter/RConn1 -- Controlled Reservoir (MA)/RConn2
  Simulink-PS Converter1/RConn1 -- Controlled Reservoir (MA)/RConn1
  Flow Rate Sensor (MA)1/RConn1 -- B/RConn1

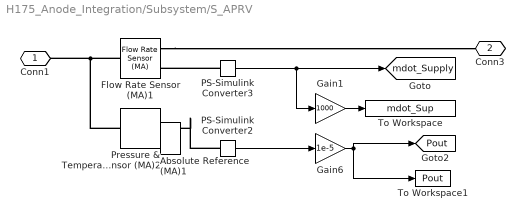
== system H175_Anode_Integration/Subsystem/S_APRV ==
  Absolute Reference (MA)1 : fl_lib/Moist Air/Elements/Absolute Reference (MA)
  Flow Rate Sensor (MA)1 : fl_lib/Moist Air/Sensors/Flow Rate Sensor (MA)  mass_flow_measure=true  volumetric_flow_measure=false  volumetric_flow_conditions=foundation.enum.volumetric_flow_conditions.actual  p_std=0.101325 MPa  T_std=20 degC  RH_std=0.65  energy_flow_measure=false  vapor_flow_measure=false  gas_flow_measure=false
      settings: LogSimulationData=on  InternalSimscapePortConfiguration="{\"Bottom\":[],\"Left\":[{\"id\":\"A\",\"label\":\"A\",\"type\":\"foundation.moist_air.moist_air\"}],\"Right\":[{\"id\":\"B\",\"label\":\"B\",\"type\":\"foundation.moist_air.moist_air\"},{\"id\":\"M\",\"label\":\"M\",\"type\":\"output\"}],\"Top\":[]}"
  Gain1 : Gain  Gain=1000
  Gain6 : Gain  Gain=1e-5
  PS-Simulink Converter2 : nesl_utility/PS-Simulink Converter  PhysicalDomain=network_engine_domain  SubClassName=ps_output  LeftPortType=input  RightPortType=output  PseudoPeriodic=off  Frequencies=[]  VectorFormat=inherit  Unit=inherit  AffineConversion=off
  PS-Simulink Converter3 : nesl_utility/PS-Simulink Converter  PhysicalDomain=network_engine_domain  SubClassName=ps_output  LeftPortType=input  RightPortType=output  PseudoPeriodic=off  Frequencies=[]  VectorFormat=inherit  Unit=inherit  AffineConversion=off
  Pressure & Temperature Sensor (MA)2 : fl_lib/Moist Air/Sensors/Pressure & Temperature Sensor (MA)  reference=foundation.enum.MeasurementReference.difference  pressure=true  pressure_spec=foundation.enum.PressureMeasementSpec.Absolute  temperature=true
      settings: InternalSimscapePortConfiguration="{\"Bottom\":[{\"id\":\"T\",\"label\":\"T\",\"type\":\"output\"}],\"Left\":[{\"id\":\"A\",\"label\":\"A\",\"type\":\"foundation.moist_air.moist_air\"}],\"Right\":[{\"id\":\"B\",\"label\":\"B\",\"type\":\"foundation.moist_air.moist_air\"},{\"id\":\"P\",\"label\":\"P\",\"type\":\"output\"}],\"Top\":[]}"
  To Workspace : ToWorkspace  VariableName=mdot_Sup  SaveFormat=Structure With Time  SampleTime=-1
  To Workspace1 : ToWorkspace  VariableName=Pout  SaveFormat=Structure With Time  SampleTime=-1
  Conn1 : PMIOPort  Side=Left
  Conn3 : PMIOPort  Port=2  Side=Right
  tag scope: Pout=global, mdot_Supply=global
  wires:
  Gain6/1 -> [Pout], To Workspace1/1
  PS-Simulink Converter3/1 -> Gain1/1, [mdot_Supply]
  PS-Simulink Converter2/1 -> Gain6/1
  Gain1/1 -> To Workspace/1
  connections:
  Flow Rate Sensor (MA)1/RConn1 -- Conn3/RConn1
  PS-Simulink Converter3/LConn1 -- Flow Rate Sensor (MA)1/RConn2
  PS-Simulink Converter2/LConn1 -- Pressure & Temperature Sensor (MA)2/RConn2
  Absolute Reference (MA)1/LConn1 -- Pressure & Temperature Sensor (MA)2/RConn1
  Flow Rate Sensor (MA)1/LConn1 -- Pressure & Temperature Sensor (MA)2/LConn1 -- Conn1/RConn1

== system H175_Anode_Integration/Subsystem/Subsystem1 ==
  PS-Simulink Converter2 : nesl_utility/PS-Simulink Converter  PhysicalDomain=network_engine_domain  SubClassName=ps_output  LeftPortType=input  RightPortType=output  PseudoPeriodic=off  Frequencies=[]  VectorFormat=inherit  Unit=inherit  AffineConversion=off
  Rec_mdot : fl_lib/Moist Air/Sensors/Flow Rate Sensor (MA)  mass_flow_measure=true  volumetric_flow_measure=false  volumetric_flow_conditions=foundation.enum.volumetric_flow_conditions.actual  p_std=0.101325 MPa  T_std=20 degC  RH_std=0.65  energy_flow_measure=false  vapor_flow_measure=true  gas_flow_measure=false
      settings: InternalSimscapePortConfiguration="{\"Bottom\":[],\"Left\":[{\"id\":\"A\",\"label\":\"A\",\"type\":\"foundation.moist_air.moist_air\"},{\"id\":\"Mw\",\"label\":\"Mw\",\"type\":\"output\"}],\"Right\":[{\"id\":\"B\",\"label\":\"B\",\"type\":\"foundation.moist_air.moist_air\"},{\"id\":\"M\",\"label\":\"M\",\"type\":\"output\"}],\"Top\":[]}"
  A : PMIOPort  Side=Left
  B : PMIOPort  Port=2  Side=Right
  tag scope: mdot_RecOut=global
  wires:
  PS-Simulink Converter2/1 -> [mdot_RecOut]
  connections:
  Rec_mdot/RConn1 -- A/RConn1
  PS-Simulink Converter2/LConn1 -- Rec_mdot/RConn2
  B/RConn1 -- Rec_mdot/LConn1

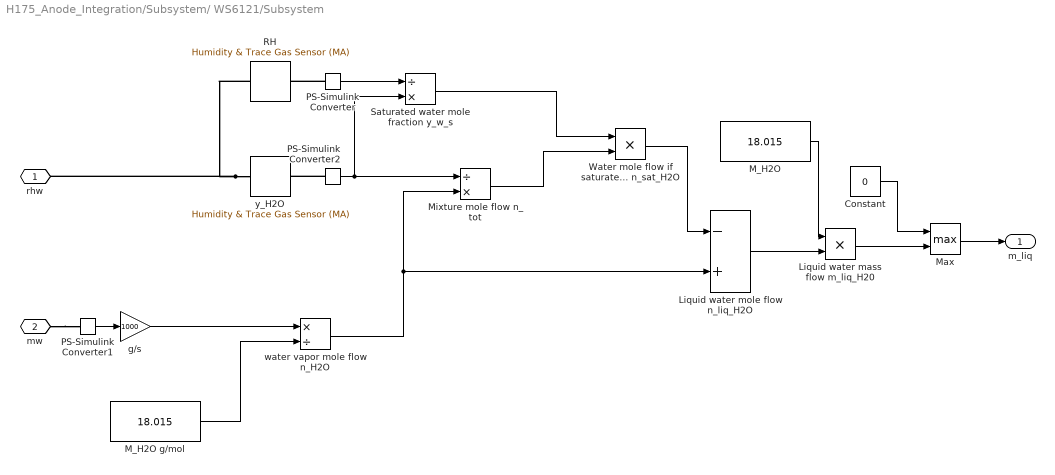
== system H175_Anode_Integration/Subsystem/ WS6121/Subsystem ==
  Constant : Constant  Value=0
  Liquid water mass flow m_liq_H20 : Product
  Liquid water mole flow n_liq_H2O : Sum  Inputs=-+
  M_H2O : Constant  Value=18.015
  M_H2O g/mol : Constant  Value=18.015
  Max : MinMax  Function=max  Inputs=2
  Mixture mole flow n_tot : Product  Inputs=/*
  PS-Simulink Converter : nesl_utility/PS-Simulink Converter  PhysicalDomain=network_engine_domain  SubClassName=ps_output  LeftPortType=input  RightPortType=output  PseudoPeriodic=off  Frequencies=[]  VectorFormat=inherit  Unit=inherit  AffineConversion=off
  PS-Simulink Converter1 : nesl_utility/PS-Simulink Converter  PhysicalDomain=network_engine_domain  SubClassName=ps_output  LeftPortType=input  RightPortType=output  PseudoPeriodic=off  Frequencies=[]  VectorFormat=inherit  Unit=inherit  AffineConversion=off
  PS-Simulink Converter2 : nesl_utility/PS-Simulink Converter  PhysicalDomain=network_engine_domain  SubClassName=ps_output  LeftPortType=input  RightPortType=output  PseudoPeriodic=off  Frequencies=[]  VectorFormat=inherit  Unit=inherit  AffineConversion=off
  RH : fl_lib/Moist Air/Sensors/Humidity & Trace Gas Sensor (MA)  moisture_on=true  moisture_spec=foundation.enum.moistureSpec.RelativeHumidity  trace_gas_on=false  trace_gas_spec=foundation.enum.trace_gas_spec.mole_fraction
      settings: InternalSimscapePortConfiguration="{\"Bottom\":[],\"Left\":[{\"id\":\"A\",\"label\":\"A\",\"type\":\"foundation.moist_air.moist_air\"}],\"Right\":[{\"id\":\"W\",\"label\":\"W\",\"type\":\"output\"}],\"Top\":[]}"
  Saturated water mole fraction y_w_s : Product  Inputs=/*
  Water mole flow if saturated n_sat_H2O : Product
  g/s : Gain  Gain=1000
  water vapor mole flow n_H2O : Product  Inputs=*/
  y_H2O : fl_lib/Moist Air/Sensors/Humidity & Trace Gas Sensor (MA)  moisture_on=true  moisture_spec=foundation.enum.moistureSpec.MoleFraction  trace_gas_on=false  trace_gas_spec=foundation.enum.trace_gas_spec.mole_fraction
      settings: InternalSimscapePortConfiguration="{\"Bottom\":[],\"Left\":[{\"id\":\"A\",\"label\":\"A\",\"type\":\"foundation.moist_air.moist_air\"}],\"Right\":[{\"id\":\"W\",\"label\":\"W\",\"type\":\"output\"}],\"Top\":[]}"
  rhw : PMIOPort  Side=Left
  mw : PMIOPort  Port=2  Side=Left
  m_liq : Outport
  wires:
  Constant/1 -> Max/1
  Max/1 -> m_liq/1
  water vapor mole flow n_H2O/1 -> Mixture mole flow n_tot/2, Liquid water mole flow n_liq_H2O/2
  PS-Simulink Converter1/1 -> g/s/1
  Liquid water mole flow n_liq_H2O/1 -> Liquid water mass flow m_liq_H20/2
  PS-Simulink Converter/1 -> Saturated water mole fraction y_w_s/1
  Liquid water mass flow m_liq_H20/1 -> Max/2
  Water mole flow if saturated n_sat_H2O/1 -> Liquid water mole flow n_liq_H2O/1
  g/s/1 -> water vapor mole flow n_H2O/1
  Saturated water mole fraction y_w_s/1 -> Water mole flow if saturated n_sat_H2O/1
  PS-Simulink Converter2/1 -> Mixture mole flow n_tot/1, Saturated water mole fraction y_w_s/2
  Mixture mole flow n_tot/1 -> Water mole flow if saturated n_sat_H2O/2
  M_H2O/1 -> Liquid water mass flow m_liq_H20/1
  M_H2O g/mol/1 -> water vapor mole flow n_H2O/2
  connections:
  y_H2O/LConn1 -- rhw/RConn1 -- RH/LConn1
  PS-Simulink Converter2/LConn1 -- y_H2O/RConn1
  PS-Simulink Converter/LConn1 -- RH/RConn1
  mw/RConn1 -- PS-Simulink Converter1/LConn1

== system H175_Anode_Integration/Subsystem/ WS6121/ValveControl ==
  Simulink-PS Converter1 : nesl_utility/Simulink-PS Converter  PhysicalDomain=network_engine_domain  SubClassName=ps_input  LeftPortType=input  RightPortType=output  PseudoPeriodic=off  Frequencies=[]  NoiseDistribution=none  NoiseParameters=[]  Unit=m^2  AffineConversion=off  FilteringAndDerivatives=provide  SimscapeFilterOrder=1  InputFilterTimeConstant=0.001  UdotUserProvided=0
  Step2 : Step  Time=10  SampleTime=0
  Transfer Fcn2 : TransferFcn  Numerator=[4.75e-6]  Denominator=[1 1]
  Cmd : PMIOPort  Side=Right
  wires:
  Transfer Fcn2/1 -> Simulink-PS Converter1/1
  Step2/1 -> Transfer Fcn2/1
  connections:
  Simulink-PS Converter1/RConn1 -- Cmd/RConn1

== matlab function H175_Anode_Integration/Anode Controller/APRV_VL6112 Valve_Control/Valve Lift Command Control ==
  data: m_dot input; p1 input; p2 input; T1 input; Kvs input; lift_signal output; rho_std input; W output
function [lift_signal,W]  = fcn(m_dot,p1,p2,T1,Kvs,rho_std)

% calculation based on Bürkert. Direktwirkendes 2-Wege-Standard-Proportionalventil. Datenblatt
% for calculation based on Swagelok. Valve Sizing. Technical Bulletin:
% check calculation_valve_formulas_comparison

% determine optimum valve opening based on pressure ratio for subscritical conditions
% Kvs - valve coefficient [m^3/h] at fully valve open
% lift_signal = Kv/Kvs (linear assumption)

dp = max(0,p1 - p2);            % avoid complex square root

% distinction of flow characteristics based on pressure drop
if p2/p1 > 0.5
    % low pressure drop - subsonic flow
    lift_signal = m_dot*3.6/(Kvs*514)*sqrt(T1/(p2*dp*rho_std));
    W=1;
  
else 
    % high pressure drop - sonic flow (independent of downstream pressure)
    %lift_signal = 0.05;
    lift_signal = m_dot*3.6/(Kvs*257*p1)*sqrt(T1/rho_std);
     W=2;
end
